simulink model "exp1_local_rendering_stg1"  (R2025a)
settings: Solver=ode4  StartTime=0.0  StopTime=2  FixedStep=1e-4  RelTol=1e-3
undefined symbols (not defined in the file or in its folder): b_eq, Bc, I_eq, k_eq, Kc, r_h, r_m, r_s, vM0, xM0
settings Model: Creator=ekaitz  LastModifiedBy=ekaitz

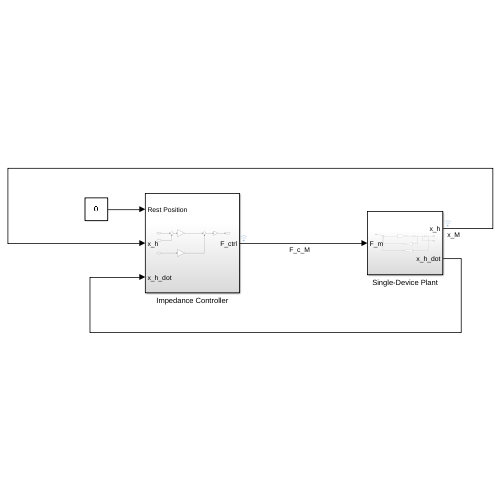
[thumbnail: Simulink's stored preview of the top-level diagram]
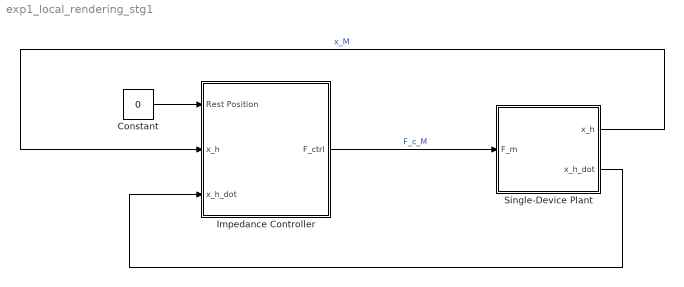
== system exp1_local_rendering_stg1 ==
  Constant : Constant  Value=0
  Impedance Controller : Subsystem
  Single-Device Plant : Subsystem
  wires:
  Single-Device Plant/1(x_h) -> Impedance Controller/2(x_h)  "x_M"
  Constant/1 -> Impedance Controller/1(Rest Position)
  Impedance Controller/1(F_ctrl) -> Single-Device Plant/1(F_m)  "F_c_M"
  Single-Device Plant/2(x_h_dot) -> Impedance Controller/3(x_h_dot)

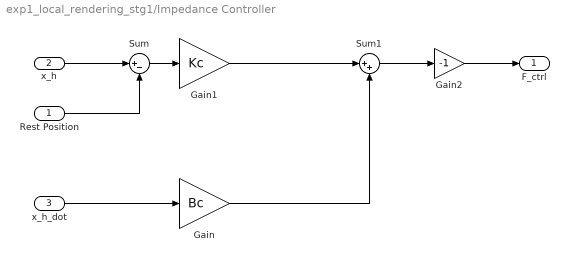
== system exp1_local_rendering_stg1/Impedance Controller ==
  Rest Position : Inport
  x_h : Inport  Port=2
  x_h_dot : Inport  Port=3
  Gain : Gain  Gain=Bc
  Gain1 : Gain  Gain=Kc
  Gain2 : Gain  Gain=-1
  Sum : Sum  Inputs=|+-
  Sum1 : Sum  Inputs=|++
  F_ctrl : Outport
  wires:
  x_h/1 -> Sum/1
  Rest Position/1 -> Sum/2
  x_h_dot/1 -> Gain/1
  Sum/1 -> Gain1/1
  Sum1/1 -> Gain2/1
  Gain1/1 -> Sum1/1
  Gain/1 -> Sum1/2
  Gain2/1 -> F_ctrl/1

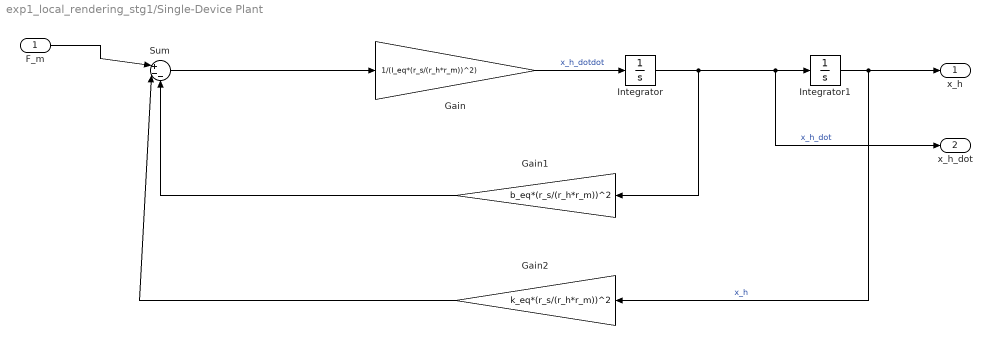
== system exp1_local_rendering_stg1/Single-Device Plant ==
  F_m : Inport
  Gain : Gain  Gain=1/(I_eq*(r_s/(r_h*r_m))^2)
  Gain1 : Gain  Gain=b_eq*(r_s/(r_h*r_m))^2
  Gain2 : Gain  Gain=k_eq*(r_s/(r_h*r_m))^2
  Integrator : Integrator  InitialCondition=vM0
  Integrator1 : Integrator  InitialCondition=xM0
  Sum : Sum  Inputs=|+--
  x_h : Outport
  x_h_dot : Outport  Port=2
  wires:
  Gain2/1 -> Sum/2
  Gain/1 -> Integrator/1  "x_h_dotdot"
  F_m/1 -> Sum/1
  Integrator1/1 -> x_h/1, Gain2/1  "x_h"
  Gain1/1 -> Sum/3
  Sum/1 -> Gain/1
  Integrator/1 -> Gain1/1, x_h_dot/1, Integrator1/1  "x_h_dot"
